simulink model "pfccontoller"  (R2023b)
settings: Solver=VariableStepAuto  StartTime=0.0  StopTime=10.0  RelTol=1e-3
values from neighbouring files (symbols this model uses):
  pfcsubsystem_data =     [pfc_controller_data.mat]    (also in pfc_data.mat; pfc_subsystem_data.mat)
undefined symbols (not defined in the file or in its folder): hasLag, InitialLongVel, NumEgoStates
libraries: mpcsigdimcheck_private x19, simulink x2, mpclib x2
settings Model: Creator=yedhukrishna  LastModifiedBy=yedhukrishna

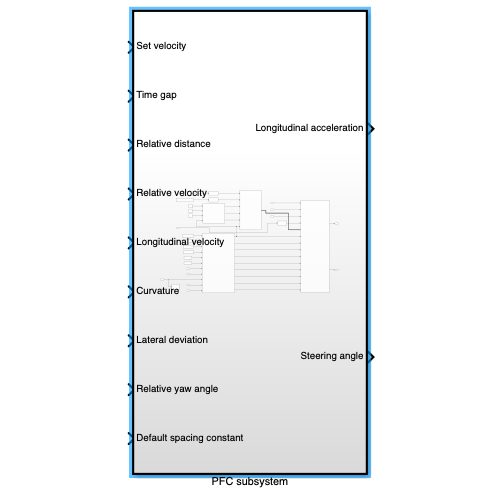
[thumbnail: Simulink's stored preview of the top-level diagram]
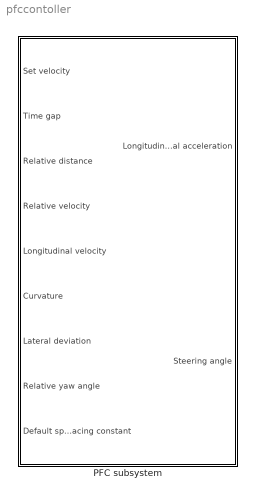
== system pfccontoller ==
  PFC subsystem : Subsystem  TreatAsAtomicUnit=on  VariantControl=Variant2
      settings: LibrarySourceBlock=mpcadaslib/Path Following Control System  RTWFileNameOpts=Use function name

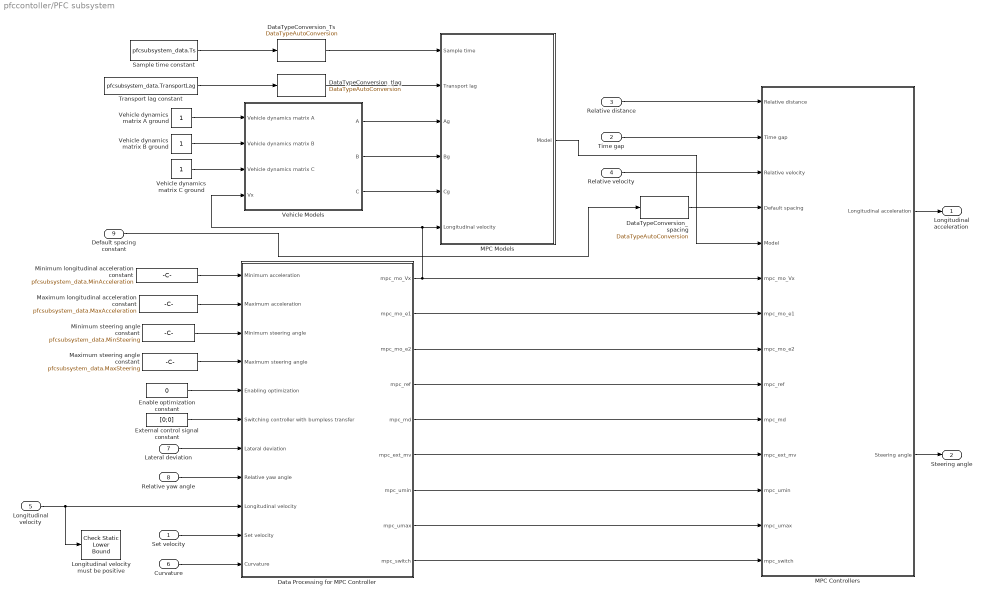
== system pfccontoller/PFC subsystem ==
  Set velocity : Inport
  Time gap : Inport  Port=2
  Relative distance : Inport  Port=3
  Relative velocity : Inport  Port=4
  Longitudinal velocity : Inport  Port=5
  Curvature : Inport  Port=6
  Lateral deviation : Inport  Port=7
  Relative yaw angle : Inport  Port=8
  Default spacing constant : Inport  Port=9
  Data Processing for MPC Controller : Subsystem
  DataTypeConversion_Ts : mpcsigdimcheck_private/DataTypeAutoConversion  datatypestr=pfcsubsystem_data.DataType
  DataTypeConversion_spacing : mpcsigdimcheck_private/DataTypeAutoConversion  datatypestr=pfcsubsystem_data.DataType
  DataTypeConversion_tlag : mpcsigdimcheck_private/DataTypeAutoConversion  datatypestr=pfcsubsystem_data.DataType
  Enable optimization constant : Constant  Value=0  OutDataTypeStr=pfcsubsystem_data.DataType
  External control signal constant : Constant  Value=[0;0]  VectorParams1D=off  OutDataTypeStr=pfcsubsystem_data.DataType
  Longitudinal velocity must be positive : simulink/Model Verification/Check Static  Lower Bound  Description=0 < u  min=0  min_included=off  enabled=on  stopWhenAssertionFail=on  export=off  icon=graphic
  MPC Controllers : Subsystem  Variant=on  VariantControlMode=label  VariantControl=Variant1  LabelModeActiveChoice=pathFollowingHasSpacingCtrl
  MPC Models : Subsystem  Variant=on  VariantControlMode=label  VariantControl=Variant1  LabelModeActiveChoice=pathFollowingHasSpacingCtrl
  Maximum longitudinal acceleration constant : Constant  Value=pfcsubsystem_data.MaxAcceleration  OutDataTypeStr=pfcsubsystem_data.DataType
  Maximum steering angle constant : Constant  Value=pfcsubsystem_data.MaxSteering  OutDataTypeStr=pfcsubsystem_data.DataType
  Minimum longitudinal acceleration constant : Constant  Value=pfcsubsystem_data.MinAcceleration  OutDataTypeStr=pfcsubsystem_data.DataType
  Minimum steering angle constant : Constant  Value=pfcsubsystem_data.MinSteering  OutDataTypeStr=pfcsubsystem_data.DataType
  Sample time constant : Constant  Value=pfcsubsystem_data.Ts  OutDataTypeStr=pfcsubsystem_data.DataType
  Transport lag constant : Constant  Value=pfcsubsystem_data.TransportLag  OutDataTypeStr=pfcsubsystem_data.DataType
  Vehicle Models : Subsystem  Variant=on  VariantControlMode=label  VariantControl=Variant1  LabelModeActiveChoice=useVehicleParameters
  Vehicle dynamics matrix A ground : Constant  OutDataTypeStr=pfcsubsystem_data.DataType
  Vehicle dynamics matrix B ground : Constant  OutDataTypeStr=pfcsubsystem_data.DataType
  Vehicle dynamics matrix C ground : Constant  OutDataTypeStr=pfcsubsystem_data.DataType
  Longitudinal acceleration : Outport  PortDimensions=1  VectorParamsAs1DForOutWhenUnconnected=off
  Steering angle : Outport  Port=2  VectorParamsAs1DForOutWhenUnconnected=off
  wires:
  MPC Controllers/1(" Longitudinal acceleration") -> Longitudinal acceleration/1
  Default spacing constant/1 -> DataTypeConversion_spacing/1
  Data Processing for MPC Controller/9(mpc_switch) -> MPC Controllers/14("mpc_switch ")
  MPC Models/1(" Model") -> MPC Controllers/5("Model ")
  Data Processing for MPC Controller/8(mpc_umax) -> MPC Controllers/13("mpc_umax ")
  MPC Controllers/2("  Steering angle") -> Steering angle/1
  Data Processing for MPC Controller/1(mpc_mo_Vx) -> MPC Controllers/6("mpc_mo_Vx "), MPC Models/6("Longitudinal velocity "), Vehicle Models/4("Vx ")
  Data Processing for MPC Controller/5(mpc_md) -> MPC Controllers/10("mpc_md ")
  Data Processing for MPC Controller/3(mpc_mo_e2) -> MPC Controllers/8("mpc_mo_e2 ")
  Data Processing for MPC Controller/4(mpc_ref) -> MPC Controllers/9("mpc_ref ")
  Longitudinal velocity/1 -> Data Processing for MPC Controller/9(Longitudinal velocity), Longitudinal velocity must be positive/1
  Data Processing for MPC Controller/2(mpc_mo_e1) -> MPC Controllers/7("mpc_mo_e1 ")
  Data Processing for MPC Controller/6(mpc_ext_mv) -> MPC Controllers/11("mpc_ext_mv ")
  Data Processing for MPC Controller/7(mpc_umin) -> MPC Controllers/12("mpc_umin ")
  Curvature/1 -> Data Processing for MPC Controller/11(Curvature)
  Set velocity/1 -> Data Processing for MPC Controller/10(Set velocity)
  Lateral deviation/1 -> Data Processing for MPC Controller/7(Lateral deviation)
  Relative yaw angle/1 -> Data Processing for MPC Controller/8(Relative yaw angle)
  Maximum longitudinal acceleration constant/1 -> Data Processing for MPC Controller/2(Maximum acceleration)
  Maximum steering angle constant/1 -> Data Processing for MPC Controller/4(Maximum steering angle)
  Enable optimization constant/1 -> Data Processing for MPC Controller/5(Enabling optimization)
  External control signal constant/1 -> Data Processing for MPC Controller/6(Switching controller with bumpless transfer)
  Minimum longitudinal acceleration constant/1 -> Data Processing for MPC Controller/1(Minimum acceleration)
  Minimum steering angle constant/1 -> Data Processing for MPC Controller/3(Minimum steering angle)
  Vehicle Models/1(" A") -> MPC Models/3(Ag)
  Vehicle Models/2(" B") -> MPC Models/4(Bg)
  Vehicle Models/3(" C") -> MPC Models/5(Cg)
  Transport lag constant/1 -> DataTypeConversion_tlag/1
  Sample time constant/1 -> DataTypeConversion_Ts/1
  Time gap/1 -> MPC Controllers/2("Time gap ")
  Relative distance/1 -> MPC Controllers/1("Relative distance ")
  Relative velocity/1 -> MPC Controllers/3("Relative velocity ")
  Vehicle dynamics matrix A ground/1 -> Vehicle Models/1(Vehicle dynamics matrix A)
  Vehicle dynamics matrix C ground/1 -> Vehicle Models/3(Vehicle dynamics matrix C)
  Vehicle dynamics matrix B ground/1 -> Vehicle Models/2(Vehicle dynamics matrix B)
  DataTypeConversion_Ts/1 -> MPC Models/1(Sample time)
  DataTypeConversion_tlag/1 -> MPC Models/2(Transport lag)
  DataTypeConversion_spacing/1 -> MPC Controllers/4("Default spacing ")

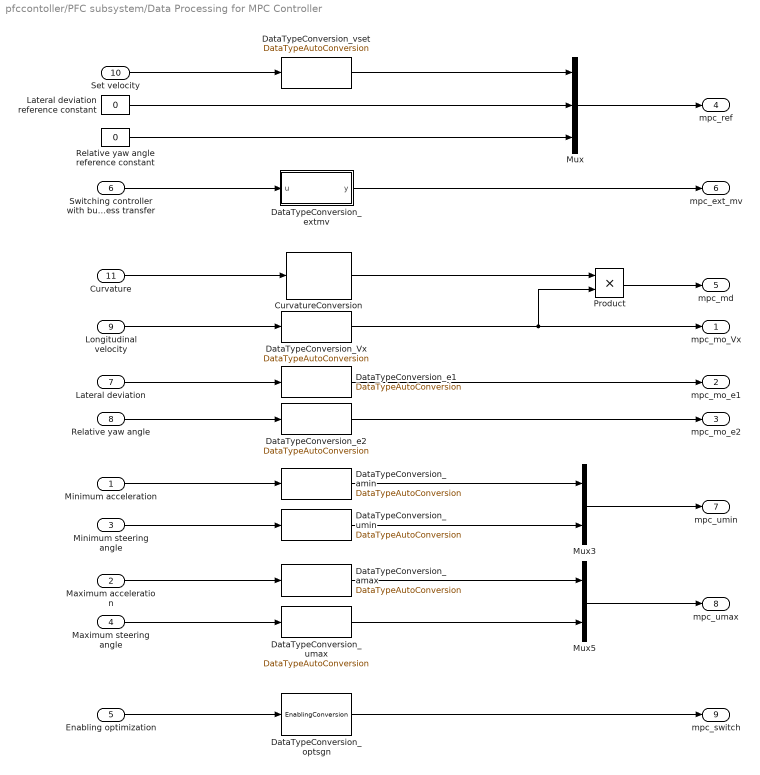
== system pfccontoller/PFC subsystem/Data Processing for MPC Controller ==
  Minimum acceleration : Inport
  Maximum acceleration : Inport  Port=2
  Minimum steering angle : Inport  Port=3
  Maximum steering angle : Inport  Port=4
  Enabling optimization : Inport  Port=5
  Switching controller with bumpless transfer : Inport  Port=6
  Lateral deviation : Inport  Port=7
  Relative yaw angle : Inport  Port=8
  Longitudinal velocity : Inport  Port=9
  Set velocity : Inport  Port=10
  Curvature : Inport  Port=11
  CurvatureConversion : mpcsigdimcheck_private/CurvatureConversion  datatypestr=pfcsubsystem_data.DataType  p=pfcsubsystem_data.Controller.PredictionHorizon
  DataTypeConversion_Vx : mpcsigdimcheck_private/DataTypeAutoConversion  datatypestr=pfcsubsystem_data.DataType
  DataTypeConversion_amax : mpcsigdimcheck_private/DataTypeAutoConversion  datatypestr=pfcsubsystem_data.DataType
  DataTypeConversion_amin : mpcsigdimcheck_private/DataTypeAutoConversion  datatypestr=pfcsubsystem_data.DataType
  DataTypeConversion_e1 : mpcsigdimcheck_private/DataTypeAutoConversion  datatypestr=pfcsubsystem_data.DataType
  DataTypeConversion_e2 : mpcsigdimcheck_private/DataTypeAutoConversion  datatypestr=pfcsubsystem_data.DataType
  DataTypeConversion_extmv : MATLAB Function  TreatAsAtomicUnit=on  mask(MPCDataTypeAutoConversion){datatypestr=pfcsubsystem_data.DataType}
      mask prompts: datatypestr "Data type"
      mask init:
      | isDouble = strcmp(datatypestr,'double');
  DataTypeConversion_optsgn : mpcsigdimcheck_private/EnablingConversion  SystemSampleTime=-1  VariantActivationTime=update diagram  AllowFlexibleInterface=on  Latency=0  AutoFrameSizeCalculation=off
  DataTypeConversion_umax : mpcsigdimcheck_private/DataTypeAutoConversion  datatypestr=pfcsubsystem_data.DataType
  DataTypeConversion_umin : mpcsigdimcheck_private/DataTypeAutoConversion  datatypestr=pfcsubsystem_data.DataType
  DataTypeConversion_vset : mpcsigdimcheck_private/DataTypeAutoConversion  datatypestr=pfcsubsystem_data.DataType
  Lateral deviation reference constant : Constant  Value=0  OutDataTypeStr=pfcsubsystem_data.DataType
  Mux : Mux  Inputs=3
  Mux3 : Mux  Inputs=2
  Mux5 : Mux  Inputs=2
  Product : Product
  "Relative yaw angle reference constant " : Constant  Value=0  OutDataTypeStr=pfcsubsystem_data.DataType
  mpc_mo_Vx : Outport  VectorParamsAs1DForOutWhenUnconnected=off
  mpc_mo_e1 : Outport  Port=2  VectorParamsAs1DForOutWhenUnconnected=off
  mpc_mo_e2 : Outport  Port=3  VectorParamsAs1DForOutWhenUnconnected=off
  mpc_ref : Outport  Port=4  VectorParamsAs1DForOutWhenUnconnected=off
  mpc_md : Outport  Port=5  VectorParamsAs1DForOutWhenUnconnected=off
  mpc_ext_mv : Outport  Port=6  VectorParamsAs1DForOutWhenUnconnected=off
  mpc_umin : Outport  Port=7  VectorParamsAs1DForOutWhenUnconnected=off
  mpc_umax : Outport  Port=8  VectorParamsAs1DForOutWhenUnconnected=off
  mpc_switch : Outport  Port=9  VectorParamsAs1DForOutWhenUnconnected=off
  wires:
  Longitudinal velocity/1 -> DataTypeConversion_Vx/1
  Curvature/1 -> CurvatureConversion/1
  Mux5/1 -> mpc_umax/1
  Lateral deviation reference constant/1 -> Mux/2
  Maximum steering angle/1 -> DataTypeConversion_umax/1
  Minimum steering angle/1 -> DataTypeConversion_umin/1
  DataTypeConversion_amin/1 -> Mux3/1
  CurvatureConversion/1 -> Product/1
  Product/1 -> mpc_md/1
  DataTypeConversion_e2/1 -> mpc_mo_e2/1
  Maximum acceleration/1 -> DataTypeConversion_amax/1
  Lateral deviation/1 -> DataTypeConversion_e1/1
  DataTypeConversion_umin/1 -> Mux3/2
  DataTypeConversion_amax/1 -> Mux5/1
  DataTypeConversion_Vx/1 -> mpc_mo_Vx/1, Product/2
  DataTypeConversion_umax/1 -> Mux5/2
  Minimum acceleration/1 -> DataTypeConversion_amin/1
  Set velocity/1 -> DataTypeConversion_vset/1
  Switching controller with bumpless transfer/1 -> DataTypeConversion_extmv/1(u)
  "Relative yaw angle reference constant "/1 -> Mux/3
  DataTypeConversion_extmv/1(y) -> mpc_ext_mv/1
  Mux3/1 -> mpc_umin/1
  Relative yaw angle/1 -> DataTypeConversion_e2/1
  DataTypeConversion_vset/1 -> Mux/1
  Mux/1 -> mpc_ref/1
  DataTypeConversion_e1/1 -> mpc_mo_e1/1
  Enabling optimization/1 -> DataTypeConversion_optsgn/1
  DataTypeConversion_optsgn/1 -> mpc_switch/1

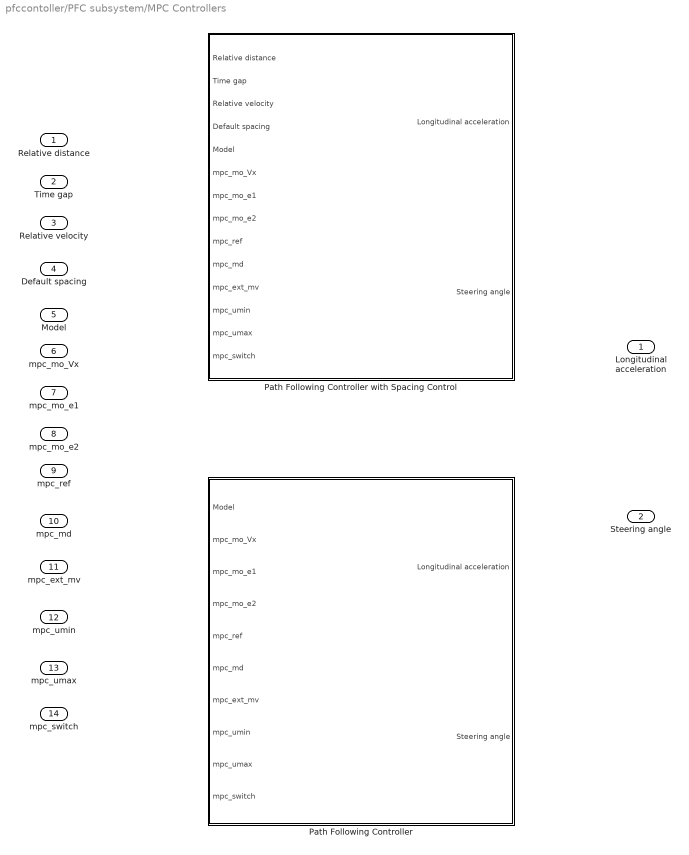
== system pfccontoller/PFC subsystem/MPC Controllers ==
  "Relative distance " : Inport
  "Time gap " : Inport  Port=2
  "Relative velocity " : Inport  Port=3
  "Default spacing " : Inport  Port=4
  "Model " : Inport  Port=5
  "mpc_mo_Vx " : Inport  Port=6
  "mpc_mo_e1 " : Inport  Port=7
  "mpc_mo_e2 " : Inport  Port=8
  "mpc_ref " : Inport  Port=9
  "mpc_md " : Inport  Port=10
  "mpc_ext_mv " : Inport  Port=11
  "mpc_umin " : Inport  Port=12
  "mpc_umax " : Inport  Port=13
  "mpc_switch " : Inport  Port=14
  Path Following Controller : Subsystem  VariantControl=pathFollowingNoSpacingCtrl
  Path Following Controller with Spacing Control : Subsystem  VariantControl=pathFollowingHasSpacingCtrl
  " Longitudinal acceleration" : Outport  VectorParamsAs1DForOutWhenUnconnected=off
  "  Steering angle" : Outport  Port=2  VectorParamsAs1DForOutWhenUnconnected=off

== system pfccontoller/PFC subsystem/MPC Models ==
  Sample time : Inport
  Transport lag : Inport  Port=2
  Ag : Inport  Port=3
  Bg : Inport  Port=4
  Cg : Inport  Port=5
  "Longitudinal velocity " : Inport  Port=6
  MPC Model : Subsystem  VariantControl=pathFollowingNoSpacingCtrl
  MPC Model with Spacing Control : Subsystem  VariantControl=pathFollowingHasSpacingCtrl
  " Model" : Outport  VectorParamsAs1DForOutWhenUnconnected=off

== system pfccontoller/PFC subsystem/Vehicle Models ==
  Vehicle dynamics matrix A : Inport
  Vehicle dynamics matrix B : Inport  Port=2
  Vehicle dynamics matrix C : Inport  Port=3
  "Vx " : Inport  Port=4
  Vehicle external model : Subsystem  VariantControl=useVehicleModel
  Vehicle parametric model : Subsystem  VariantControl=useVehicleParameters
  " A" : Outport  VectorParamsAs1DForOutWhenUnconnected=off
  " B" : Outport  Port=2  VectorParamsAs1DForOutWhenUnconnected=off
  " C" : Outport  Port=3  VectorParamsAs1DForOutWhenUnconnected=off

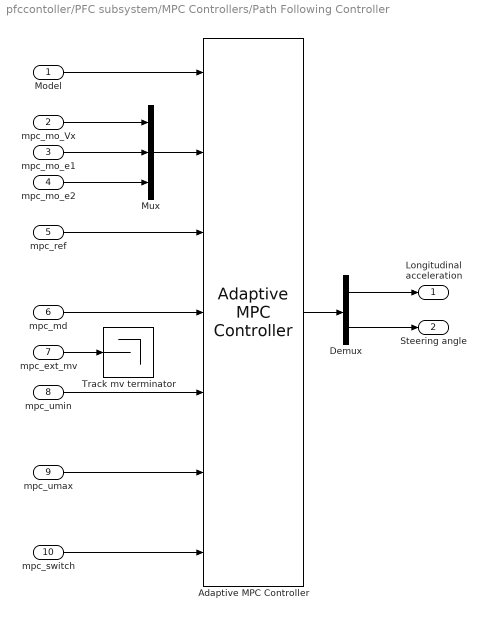
== system pfccontoller/PFC subsystem/MPC Controllers/Path Following Controller ==
  Model : Inport
  mpc_mo_Vx : Inport  Port=2
  mpc_mo_e1 : Inport  Port=3
  mpc_mo_e2 : Inport  Port=4
  mpc_ref : Inport  Port=5
  mpc_md : Inport  Port=6
  mpc_ext_mv : Inport  Port=7
  mpc_umin : Inport  Port=8
  mpc_umax : Inport  Port=9
  mpc_switch : Inport  Port=10
  Adaptive MPC Controller : mpclib/Adaptive MPC Controller  SCDEnableBlockLinearizationSpecification=on  mpcobj=mpcobj  enable_value=0  updateMPCinCallerWorkspace=off  md_inport=on  mv_inport=off  uref_inport=off  return_cost=off  return_mvseq=off  return_qpstatus=off  return_xseq=off  return_state=off  return_ovseq=off  state_inport=off  isltv_plant=off  umin_inport=on  umax_inport=on  ymin_inport=off  ymax_inport=off  cc_inport=off  ywt_inport=off  uwt_inport=off  duwt_inport=off  rhoeps_inport=off  pm_inport=off  MaximumP=10  HorizonChoice=FixedHorizon  BlockDataType=double  SampleTimeInherited=off  switch_inport=on
  Demux : Demux  Outputs=2
  Mux : Mux  Inputs=3
  Track mv terminator : Terminator
  Longitudinal acceleration : Outport  Unit=m/s^2  VectorParamsAs1DForOutWhenUnconnected=off
  " Steering angle" : Outport  Port=2  Unit=rad  VectorParamsAs1DForOutWhenUnconnected=off
  wires:
  mpc_mo_Vx/1 -> Mux/1
  Adaptive MPC Controller/1 -> Demux/1
  Mux/1 -> Adaptive MPC Controller/2
  Model/1 -> Adaptive MPC Controller/1
  mpc_mo_e2/1 -> Mux/3
  mpc_mo_e1/1 -> Mux/2
  mpc_ref/1 -> Adaptive MPC Controller/3
  mpc_md/1 -> Adaptive MPC Controller/4
  mpc_umax/1 -> Adaptive MPC Controller/6
  mpc_umin/1 -> Adaptive MPC Controller/5
  mpc_switch/1 -> Adaptive MPC Controller/7
  Demux/1 -> Longitudinal acceleration/1
  Demux/2 -> " Steering angle"/1
  mpc_ext_mv/1 -> Track mv terminator/1

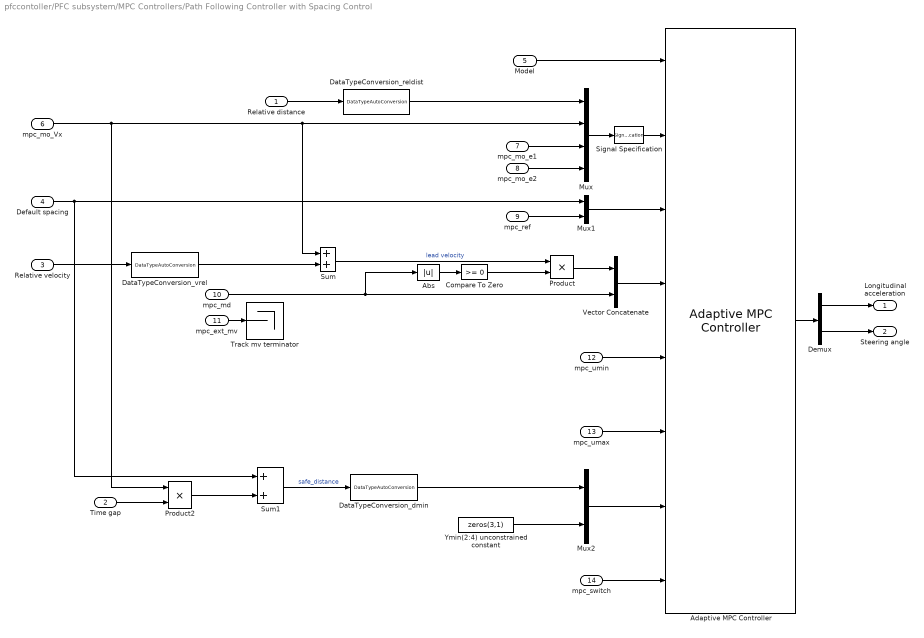
== system pfccontoller/PFC subsystem/MPC Controllers/Path Following Controller with Spacing Control ==
  Relative distance : Inport  Unit=m
  Time gap : Inport  Port=2
  Relative velocity : Inport  Port=3  Unit=m/s
  Default spacing : Inport  Port=4
  Model : Inport  Port=5
  mpc_mo_Vx : Inport  Port=6
  mpc_mo_e1 : Inport  Port=7
  mpc_mo_e2 : Inport  Port=8
  mpc_ref : Inport  Port=9
  mpc_md : Inport  Port=10
  mpc_ext_mv : Inport  Port=11
  mpc_umin : Inport  Port=12
  mpc_umax : Inport  Port=13
  mpc_switch : Inport  Port=14
  Abs : Abs  ZeroCross=off  SaturateOnIntegerOverflow=off
  Adaptive MPC Controller : mpclib/Adaptive MPC Controller  SCDEnableBlockLinearizationSpecification=on  mpcobj=pfcsubsystem_data.Controller  enable_value=0  updateMPCinCallerWorkspace=off  md_inport=on  mv_inport=off  uref_inport=off  return_cost=off  return_mvseq=off  return_qpstatus=off  return_xseq=off  return_state=off  return_ovseq=off  state_inport=off  isltv_plant=off  umin_inport=on  umax_inport=on  ymin_inport=on  ymax_inport=off  cc_inport=off  ywt_inport=off  uwt_inport=off  duwt_inport=off  rhoeps_inport=off  pm_inport=off  MaximumP=10  HorizonChoice=FixedHorizon  BlockDataType=double  SampleTimeInherited=off  switch_inport=on
  Compare To Zero : simulink/Logic and Bit Operations/Compare To Zero  relop=>=  OutDataTypeStr=boolean  ZeroCross=off
  DataTypeConversion_dmin : mpcsigdimcheck_private/DataTypeAutoConversion  datatypestr=pfcsubsystem_data.DataType
  DataTypeConversion_reldist : mpcsigdimcheck_private/DataTypeAutoConversion  datatypestr=pfcsubsystem_data.DataType
  DataTypeConversion_vrel : mpcsigdimcheck_private/DataTypeAutoConversion  datatypestr=pfcsubsystem_data.DataType
  Demux : Demux  Outputs=2
  Mux : Mux
  Mux1 : Mux  Inputs=2
  Mux2 : Mux  Inputs=2
  Product : Product
  Product2 : Product
  Signal Specification : SignalSpecification  Dimensions=4
  Sum : Sum
  Sum1 : Sum
  Track mv terminator : Terminator
  Vector Concatenate : Concatenate  Mode=Multidimensional array  ConcatenateDimension=2
  Ymin(2:4) unconstrained constant : Constant  Value=zeros(3,1)  VectorParams1D=off  OutDataTypeStr=pfcsubsystem_data.DataType
  Longitudinal acceleration : Outport  Unit=m/s^2  VectorParamsAs1DForOutWhenUnconnected=off
  " Steering angle" : Outport  Port=2  Unit=rad  VectorParamsAs1DForOutWhenUnconnected=off
  wires:
  Mux2/1 -> Adaptive MPC Controller/7
  Ymin(2:4) unconstrained constant/1 -> Mux2/2
  DataTypeConversion_reldist/1 -> Mux/1
  mpc_umin/1 -> Adaptive MPC Controller/5
  Demux/1 -> Longitudinal acceleration/1
  Model/1 -> Adaptive MPC Controller/1
  mpc_mo_e2/1 -> Mux/4
  Mux/1 -> Signal Specification/1
  Default spacing/1 -> Mux1/1, Sum1/1
  Relative velocity/1 -> DataTypeConversion_vrel/1
  mpc_mo_Vx/1 -> Product2/1, Mux/2, Sum/1
  mpc_umax/1 -> Adaptive MPC Controller/6
  Mux1/1 -> Adaptive MPC Controller/3
  Relative distance/1 -> DataTypeConversion_reldist/1
  Product2/1 -> Sum1/2
  mpc_switch/1 -> Adaptive MPC Controller/8
  Adaptive MPC Controller/1 -> Demux/1
  mpc_mo_e1/1 -> Mux/3
  Time gap/1 -> Product2/2
  Sum1/1 -> DataTypeConversion_dmin/1  "safe_distance"
  Sum/1 -> Product/1  "lead velocity"
  Demux/2 -> " Steering angle"/1
  DataTypeConversion_dmin/1 -> Mux2/1
  Signal Specification/1 -> Adaptive MPC Controller/2
  Vector Concatenate/1 -> Adaptive MPC Controller/4
  mpc_ref/1 -> Mux1/2
  mpc_ext_mv/1 -> Track mv terminator/1
  DataTypeConversion_vrel/1 -> Sum/2
  Abs/1 -> Compare To Zero/1
  mpc_md/1 -> Abs/1, Vector Concatenate/2
  Compare To Zero/1 -> Product/2
  Product/1 -> Vector Concatenate/1

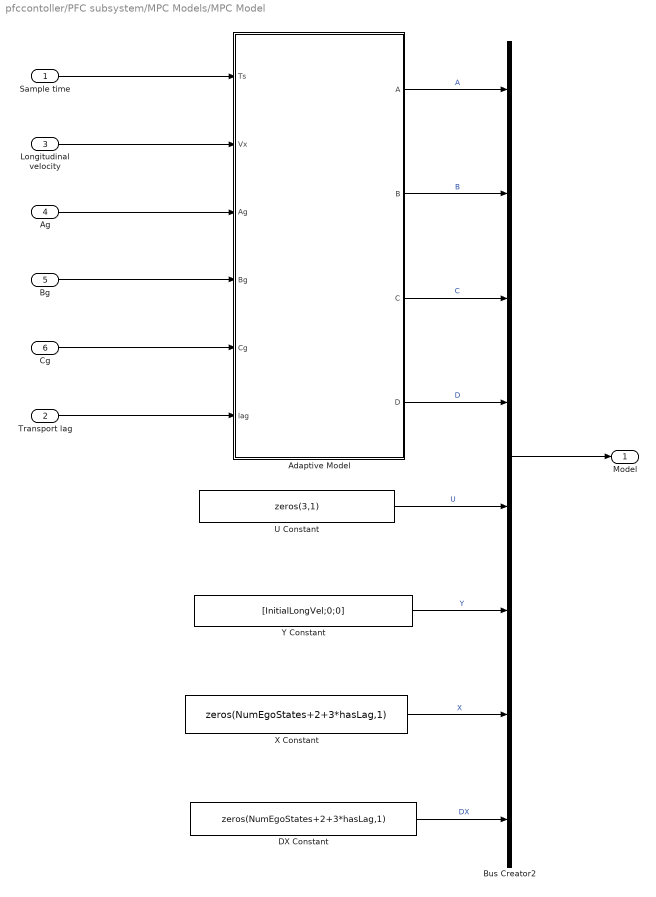
== system pfccontoller/PFC subsystem/MPC Models/MPC Model ==
  Sample time : Inport
  Transport lag : Inport  Port=2
  Longitudinal velocity : Inport  Port=3
  Ag : Inport  Port=4
  Bg : Inport  Port=5
  Cg : Inport  Port=6
  Adaptive Model : MATLAB Function  TreatAsAtomicUnit=on
  Bus Creator2 : BusCreator  Inputs=8
  DX Constant : Constant  Value=zeros(NumEgoStates+2+3*hasLag,1)  VectorParams1D=off  OutDataTypeStr=pfcsubsystem_data.DataType
  U Constant : Constant  Value=zeros(3,1)  VectorParams1D=off  OutDataTypeStr=pfcsubsystem_data.DataType
  X Constant : Constant  Value=zeros(NumEgoStates+2+3*hasLag,1)  VectorParams1D=off  OutDataTypeStr=pfcsubsystem_data.DataType
  Y Constant : Constant  Value=[InitialLongVel;0;0]  VectorParams1D=off  OutDataTypeStr=pfcsubsystem_data.DataType
  Model : Outport  VectorParamsAs1DForOutWhenUnconnected=off
  wires:
  Adaptive Model/2(B) -> Bus Creator2/2  "B"
  Transport lag/1 -> Adaptive Model/6(lag)
  U Constant/1 -> Bus Creator2/5  "U"
  DX Constant/1 -> Bus Creator2/8  "DX"
  Adaptive Model/3(C) -> Bus Creator2/3  "C"
  Adaptive Model/4(D) -> Bus Creator2/4  "D"
  Longitudinal velocity/1 -> Adaptive Model/2(Vx)
  Adaptive Model/1(A) -> Bus Creator2/1  "A"
  Sample time/1 -> Adaptive Model/1(Ts)
  Y Constant/1 -> Bus Creator2/6  "Y"
  X Constant/1 -> Bus Creator2/7  "X"
  Bus Creator2/1 -> Model/1
  Ag/1 -> Adaptive Model/3(Ag)
  Bg/1 -> Adaptive Model/4(Bg)
  Cg/1 -> Adaptive Model/5(Cg)

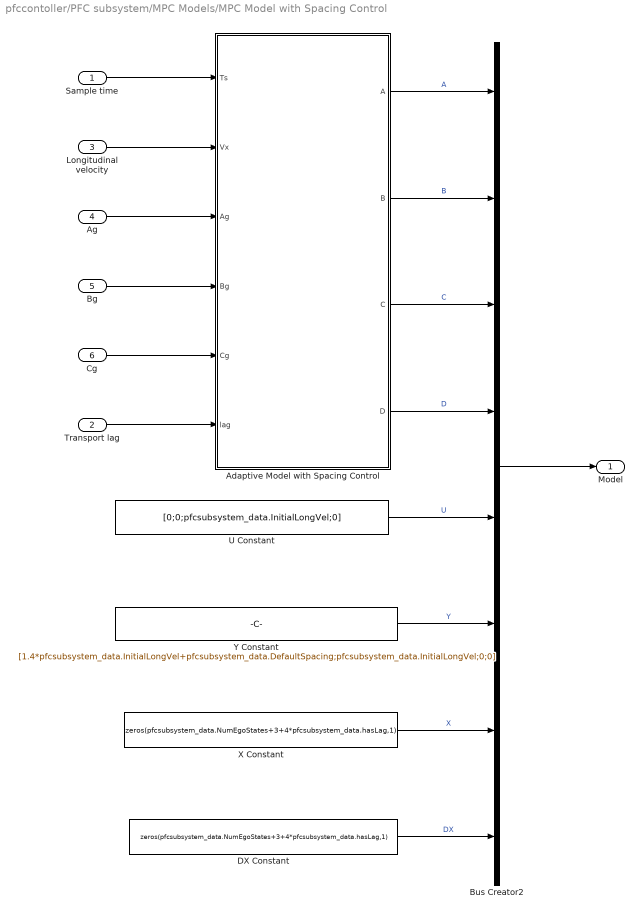
== system pfccontoller/PFC subsystem/MPC Models/MPC Model with Spacing Control ==
  Sample time : Inport
  Transport lag : Inport  Port=2
  Longitudinal velocity : Inport  Port=3
  Ag : Inport  Port=4
  Bg : Inport  Port=5
  Cg : Inport  Port=6
  Adaptive Model with Spacing Control : MATLAB Function  TreatAsAtomicUnit=on
  Bus Creator2 : BusCreator  Inputs=8
  DX Constant : Constant  Value=zeros(pfcsubsystem_data.NumEgoStates+3+4*pfcsubsystem_data.hasLag,1)  VectorParams1D=off  OutDataTypeStr=pfcsubsystem_data.DataType
  U Constant : Constant  Value=[0;0;pfcsubsystem_data.InitialLongVel;0]  VectorParams1D=off  OutDataTypeStr=pfcsubsystem_data.DataType
  X Constant : Constant  Value=zeros(pfcsubsystem_data.NumEgoStates+3+4*pfcsubsystem_data.hasLag,1)  VectorParams1D=off  OutDataTypeStr=pfcsubsystem_data.DataType
  Y Constant : Constant  Value=[1.4*pfcsubsystem_data.InitialLongVel+pfcsubsystem_data.DefaultSpacing;pfcsubsystem_data.InitialLongVel;0;0]  VectorParams1D=off  OutDataTypeStr=pfcsubsystem_data.DataType
  Model : Outport  VectorParamsAs1DForOutWhenUnconnected=off
  wires:
  Adaptive Model with Spacing Control/4(D) -> Bus Creator2/4  "D"
  X Constant/1 -> Bus Creator2/7  "X"
  Bus Creator2/1 -> Model/1
  Sample time/1 -> Adaptive Model with Spacing Control/1(Ts)
  Adaptive Model with Spacing Control/1(A) -> Bus Creator2/1  "A"
  DX Constant/1 -> Bus Creator2/8  "DX"
  Adaptive Model with Spacing Control/2(B) -> Bus Creator2/2  "B"
  Adaptive Model with Spacing Control/3(C) -> Bus Creator2/3  "C"
  Longitudinal velocity/1 -> Adaptive Model with Spacing Control/2(Vx)
  Y Constant/1 -> Bus Creator2/6  "Y"
  U Constant/1 -> Bus Creator2/5  "U"
  Ag/1 -> Adaptive Model with Spacing Control/3(Ag)
  Bg/1 -> Adaptive Model with Spacing Control/4(Bg)
  Cg/1 -> Adaptive Model with Spacing Control/5(Cg)
  Transport lag/1 -> Adaptive Model with Spacing Control/6(lag)

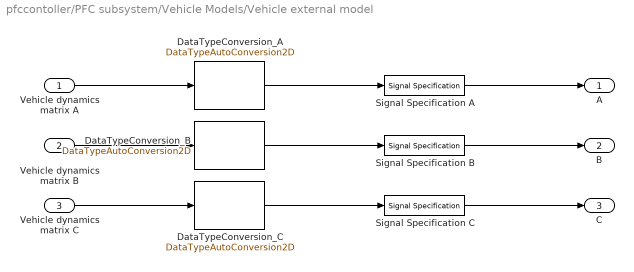
== system pfccontoller/PFC subsystem/Vehicle Models/Vehicle external model ==
  Vehicle dynamics matrix A : Inport
  Vehicle dynamics matrix B : Inport  Port=2
  Vehicle dynamics matrix C : Inport  Port=3
  DataTypeConversion_A : mpcsigdimcheck_private/DataTypeAutoConversion2D  datatypestr=pfcsubsystem_data.DataType
  DataTypeConversion_B : mpcsigdimcheck_private/DataTypeAutoConversion2D  datatypestr=pfcsubsystem_data.DataType
  DataTypeConversion_C : mpcsigdimcheck_private/DataTypeAutoConversion2D  datatypestr=pfcsubsystem_data.DataType
  Signal Specification A : SignalSpecification
  Signal Specification B : SignalSpecification
  Signal Specification C : SignalSpecification
  A : Outport  VectorParamsAs1DForOutWhenUnconnected=off
  B : Outport  Port=2  VectorParamsAs1DForOutWhenUnconnected=off
  C : Outport  Port=3  VectorParamsAs1DForOutWhenUnconnected=off
  wires:
  Signal Specification B/1 -> B/1
  Signal Specification C/1 -> C/1
  DataTypeConversion_C/1 -> Signal Specification C/1
  Signal Specification A/1 -> A/1
  Vehicle dynamics matrix A/1 -> DataTypeConversion_A/1
  Vehicle dynamics matrix C/1 -> DataTypeConversion_C/1
  DataTypeConversion_A/1 -> Signal Specification A/1
  Vehicle dynamics matrix B/1 -> DataTypeConversion_B/1
  DataTypeConversion_B/1 -> Signal Specification B/1

== system pfccontoller/PFC subsystem/Vehicle Models/Vehicle parametric model ==
  Vx : Inport
  Vehicle combined dynamics : Subsystem
  Vehicle lateral dynamics : Subsystem
  Vehicle longitudinal dynamics : Subsystem
  A : Outport  VectorParamsAs1DForOutWhenUnconnected=off
  B : Outport  Port=2  VectorParamsAs1DForOutWhenUnconnected=off
  C : Outport  Port=3  VectorParamsAs1DForOutWhenUnconnected=off
  wires:
  Vehicle combined dynamics/3(C) -> C/1
  Vehicle combined dynamics/1(A) -> A/1
  Vehicle combined dynamics/2(B) -> B/1
  Vehicle lateral dynamics/1(Am) -> Vehicle combined dynamics/4(A2)
  Vehicle lateral dynamics/2(Bm) -> Vehicle combined dynamics/5(B2)
  Vehicle lateral dynamics/3(Cm) -> Vehicle combined dynamics/6(C2)
  Vehicle longitudinal dynamics/1(An) -> Vehicle combined dynamics/1(A1)
  Vehicle longitudinal dynamics/2(Bn) -> Vehicle combined dynamics/2(B1)
  Vehicle longitudinal dynamics/3(Cn) -> Vehicle combined dynamics/3(C1)
  Vx/1 -> Vehicle lateral dynamics/1(Vx)

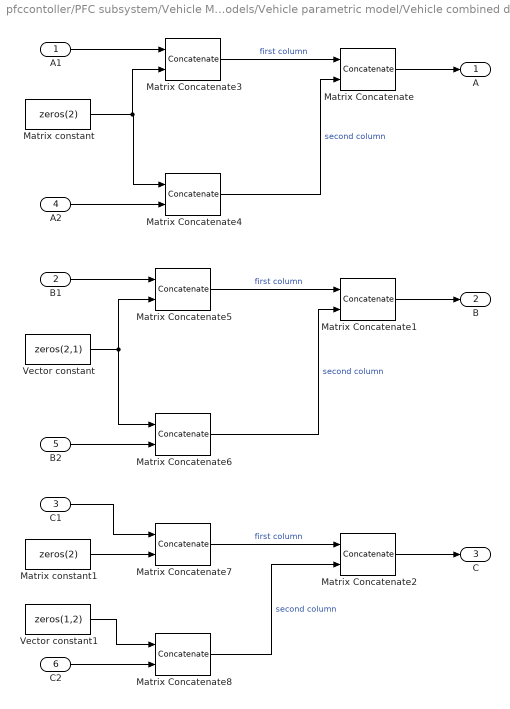
== system pfccontoller/PFC subsystem/Vehicle Models/Vehicle parametric model/Vehicle combined dynamics ==
  A1 : Inport
  B1 : Inport  Port=2
  C1 : Inport  Port=3
  A2 : Inport  Port=4
  B2 : Inport  Port=5
  C2 : Inport  Port=6
  Matrix Concatenate : Concatenate  Mode=Multidimensional array  ConcatenateDimension=2
  Matrix Concatenate1 : Concatenate  Mode=Multidimensional array  ConcatenateDimension=2
  Matrix Concatenate2 : Concatenate  Mode=Multidimensional array  ConcatenateDimension=2
  Matrix Concatenate{3..8} (6 alike) : Concatenate  Mode=Multidimensional array
  Matrix constant : Constant  Value=zeros(2)  VectorParams1D=off  OutDataTypeStr=pfcsubsystem_data.DataType
  Matrix constant1 : Constant  Value=zeros(2)  VectorParams1D=off  OutDataTypeStr=pfcsubsystem_data.DataType
  Vector constant : Constant  Value=zeros(2,1)  VectorParams1D=off  OutDataTypeStr=pfcsubsystem_data.DataType
  Vector constant1 : Constant  Value=zeros(1,2)  VectorParams1D=off  OutDataTypeStr=pfcsubsystem_data.DataType
  A : Outport  VectorParamsAs1DForOutWhenUnconnected=off
  B : Outport  Port=2  VectorParamsAs1DForOutWhenUnconnected=off
  C : Outport  Port=3  VectorParamsAs1DForOutWhenUnconnected=off
  wires:
  Vector constant/1 -> Matrix Concatenate6/1, Matrix Concatenate5/2
  C1/1 -> Matrix Concatenate7/1
  Matrix Concatenate6/1 -> Matrix Concatenate1/2  "second column"
  Matrix Concatenate4/1 -> Matrix Concatenate/2  "second column"
  B1/1 -> Matrix Concatenate5/1
  Matrix Concatenate1/1 -> B/1
  Vector constant1/1 -> Matrix Concatenate8/1
  Matrix Concatenate/1 -> A/1
  Matrix constant/1 -> Matrix Concatenate4/1, Matrix Concatenate3/2
  Matrix Concatenate2/1 -> C/1
  Matrix constant1/1 -> Matrix Concatenate7/2
  Matrix Concatenate8/1 -> Matrix Concatenate2/2  "second column"
  Matrix Concatenate7/1 -> Matrix Concatenate2/1  "first column"
  C2/1 -> Matrix Concatenate8/2
  B2/1 -> Matrix Concatenate6/2
  A2/1 -> Matrix Concatenate4/2
  Matrix Concatenate3/1 -> Matrix Concatenate/1  "first column"
  A1/1 -> Matrix Concatenate3/1
  Matrix Concatenate5/1 -> Matrix Concatenate1/1  "first column"

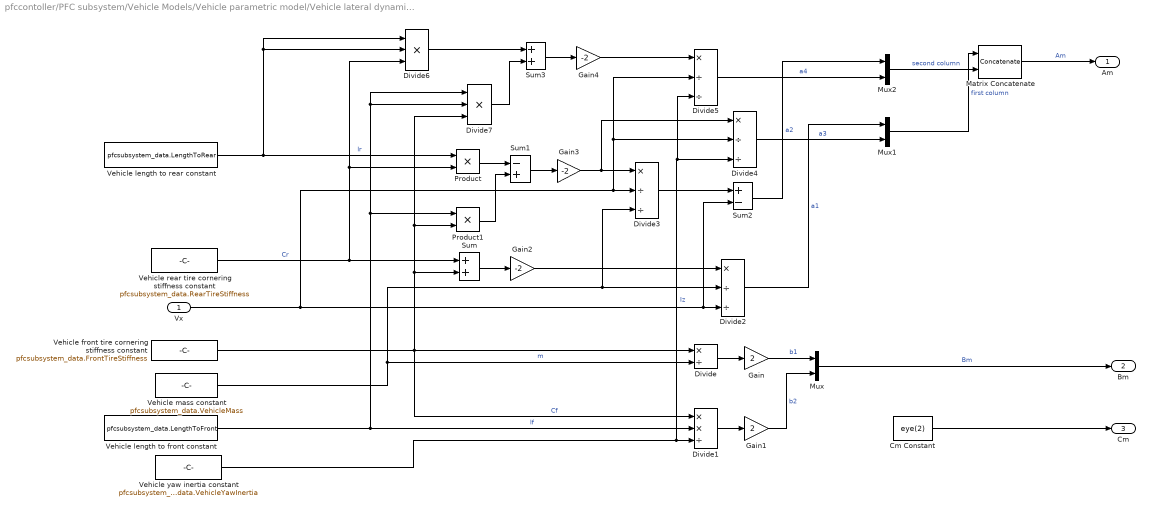
== system pfccontoller/PFC subsystem/Vehicle Models/Vehicle parametric model/Vehicle lateral dynamics ==
  Vx : Inport
  Cm Constant : Constant  Value=eye(2)  OutDataTypeStr=pfcsubsystem_data.DataType
  Divide : Product  Inputs=*/
  Divide1 : Product  Inputs=**/
  Divide{2..5} (4 alike) : Product  Inputs=*//
  Divide6 : Product  Inputs=***
  Divide7 : Product  Inputs=***
  Gain : Gain  Gain=2
  Gain1 : Gain  Gain=2
  Gain2 : Gain  Gain=-2
  Gain3 : Gain  Gain=-2
  Gain4 : Gain  Gain=-2
  Matrix Concatenate : Concatenate  Mode=Multidimensional array  ConcatenateDimension=2
  Mux : Mux  Inputs=[1 1]
  Mux1 : Mux  Inputs=[1 1]
  Mux2 : Mux  Inputs=[1 1]
  Product : Product
  Product1 : Product
  Sum : Sum
  Sum1 : Sum  Inputs=-+
  Sum2 : Sum  Inputs=+-
  Sum3 : Sum
  Vehicle front tire cornering stiffness constant : Constant  Value=pfcsubsystem_data.FrontTireStiffness  OutDataTypeStr=pfcsubsystem_data.DataType
  Vehicle length to front constant : Constant  Value=pfcsubsystem_data.LengthToFront  OutDataTypeStr=pfcsubsystem_data.DataType
  Vehicle length to rear constant : Constant  Value=pfcsubsystem_data.LengthToRear  OutDataTypeStr=pfcsubsystem_data.DataType
  Vehicle mass constant : Constant  Value=pfcsubsystem_data.VehicleMass  OutDataTypeStr=pfcsubsystem_data.DataType
  Vehicle rear tire cornering stiffness constant : Constant  Value=pfcsubsystem_data.RearTireStiffness  OutDataTypeStr=pfcsubsystem_data.DataType
  Vehicle yaw inertia constant : Constant  Value=pfcsubsystem_data.VehicleYawInertia  OutDataTypeStr=pfcsubsystem_data.DataType
  Am : Outport  VectorParamsAs1DForOutWhenUnconnected=off
  Bm : Outport  Port=2  VectorParamsAs1DForOutWhenUnconnected=off
  Cm : Outport  Port=3  VectorParamsAs1DForOutWhenUnconnected=off
  wires:
  Divide5/1 -> Mux2/2  "a4"
  Vehicle length to front constant/1 -> Divide7/1, Divide7/2, Product1/1, Divide1/2  "lf"
  Mux2/1 -> Matrix Concatenate/2  "second column"
  Product1/1 -> Sum1/2
  Vehicle front tire cornering stiffness constant/1 -> Divide1/1, Divide/1, Divide7/3, Product1/2, Sum/2  "Cf"
  Vehicle yaw inertia constant/1 -> Divide5/3, Divide4/3, Divide1/3  "Iz"
  Vehicle mass constant/1 -> Divide/2, Divide3/3, Divide2/2  "m"
  Gain4/1 -> Divide5/1
  Vehicle length to rear constant/1 -> Divide6/2, Divide6/1, Product/1  "lr"
  Vehicle rear tire cornering stiffness constant/1 -> Divide6/3, Product/2, Sum/1  "Cr"
  Sum2/1 -> Mux2/1  "a2"
  Vx/1 -> Divide3/2, Divide5/2, Divide4/2, Sum2/2, Divide2/3
  Gain/1 -> Mux/1  "b1"
  Divide2/1 -> Mux1/1  "a1"
  Product/1 -> Sum1/1
  Mux/1 -> Bm/1  "Bm"
  Divide4/1 -> Mux1/2  "a3"
  Divide7/1 -> Sum3/2
  Matrix Concatenate/1 -> Am/1  "Am"
  Sum3/1 -> Gain4/1
  Gain3/1 -> Divide3/1, Divide4/1
  Sum1/1 -> Gain3/1
  Mux1/1 -> Matrix Concatenate/1  "first column"
  Sum/1 -> Gain2/1
  Divide3/1 -> Sum2/1
  Gain1/1 -> Mux/2  "b2"
  Divide/1 -> Gain/1
  Divide1/1 -> Gain1/1
  Cm Constant/1 -> Cm/1
  Gain2/1 -> Divide2/1
  Divide6/1 -> Sum3/1

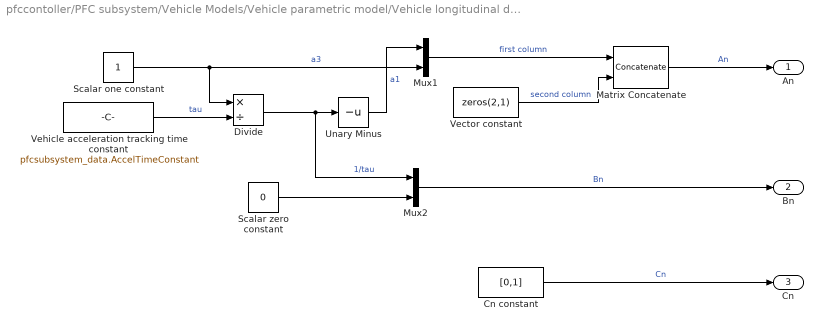
== system pfccontoller/PFC subsystem/Vehicle Models/Vehicle parametric model/Vehicle longitudinal dynamics ==
  Cn constant : Constant  Value=[0,1]  VectorParams1D=off  OutDataTypeStr=pfcsubsystem_data.DataType
  Divide : Product  Inputs=*/
  Matrix Concatenate : Concatenate  Mode=Multidimensional array  ConcatenateDimension=2
  Mux1 : Mux  Inputs=[1 1]
  Mux2 : Mux  Inputs=[1 1]
  Scalar one constant : Constant  OutDataTypeStr=pfcsubsystem_data.DataType
  Scalar zero constant : Constant  Value=0  OutDataTypeStr=pfcsubsystem_data.DataType
  Unary Minus : UnaryMinus
  Vector constant : Constant  Value=zeros(2,1)  VectorParams1D=off  OutDataTypeStr=pfcsubsystem_data.DataType
  Vehicle acceleration tracking time constant : Constant  Value=pfcsubsystem_data.AccelTimeConstant  OutDataTypeStr=pfcsubsystem_data.DataType
  An : Outport  VectorParamsAs1DForOutWhenUnconnected=off
  Bn : Outport  Port=2  VectorParamsAs1DForOutWhenUnconnected=off
  Cn : Outport  Port=3  VectorParamsAs1DForOutWhenUnconnected=off
  wires:
  Vehicle acceleration tracking time constant/1 -> Divide/2  "tau"
  Divide/1 -> Mux2/1, Unary Minus/1  "1/tau"
  Vector constant/1 -> Matrix Concatenate/2  "second column"
  Matrix Concatenate/1 -> An/1  "An"
  Cn constant/1 -> Cn/1  "Cn"
  Unary Minus/1 -> Mux1/1  "a1"
  Scalar one constant/1 -> Mux1/2, Divide/1  "a3"
  Mux2/1 -> Bn/1  "Bn"
  Scalar zero constant/1 -> Mux2/2
  Mux1/1 -> Matrix Concatenate/1  "first column"

== matlab function pfccontoller/PFC subsystem/MPC Models/MPC Model/Adaptive Model ==
  data: Ts input; A output; Vx input; Ag input; Bg input; Cg input; lag input; B output; C output; D output
function [A,B,C,D] = getAdaptiveMPCModel(Ts,Vx, Ag, Bg, Cg, lag)
% Get discrete state-space model for Adaptive MPC with sample time Ts.
% Called by the 'Path Following Control System' Block.

% Inputs:
%   Ts:               mask variable for sample time
%   Vx:               mask inport for longitudinal velocity
%   Ag,Bg,Cg:         continuous or discrete vehicle model with sample time Ts
% Outputs:
%   A,B,C,D:          discrete time model for adaptive MPC

%   Author: Meng Xia, Rong Chen
%   Copyright 2017-2018 The MathWorks, Inc.

% Discrete MPC model
[A,B,C,D] = pfcblock_utilGetDTModelHasLagForMPCNoSpacingCtrl(Ts,Vx,Ag,Bg,Cg,lag);

== matlab function pfccontoller/PFC subsystem/MPC Models/MPC Model with Spacing Control/Adaptive Model with Spacing Control ==
  data: Ts input; A output; Vx input; Ag input; Bg input; Cg input; lag input; B output; C output; D output
function [A,B,C,D] = getAdaptiveMPCModel(Ts,Vx, Ag, Bg, Cg, lag)
% Get discrete state-space model for Adaptive MPC with sample time Ts.
% Called by the 'Path Following Control System' Block.

% Inputs:
%   Ts:               mask variable for sample time
%   Vx:               mask inport for longitudinal velocity
%   Ag,Bg,Cg:         continuous or discrete vehicle model with sample time Ts
% Outputs:
%   A,B,C,D:          discrete time model for adaptive MPC

%   Author: Meng Xia, Rong Chen
%   Copyright 2017-2018 The MathWorks, Inc.

% Discrete MPC model
[A,B,C,D] = pfcblock_utilGetDTModelHasLagForMPCHasSpacingCtrl(Ts,Vx,Ag,Bg,Cg,lag);

== matlab function pfccontoller/PFC subsystem/Data Processing for MPC Controller/DataTypeConversion_extmv ==
  data: u input size=[2 1]; y output; isDouble parameter
function y = fcn(u,isDouble)
if isDouble
    if isa(u,'double')
        y = u;
    else
        y = double(u);
    end
else
    if isa(u,'single')
        y = u;
    else
        y = single(u);
    end
end
